simulink model "SALTStabilizationInnerOuterLoop"  (Simulink 7.8)
settings: Solver=FixedStepDiscrete  StartTime=0.0  StopTime=5.695  FixedStep=.001  RelTol=1e-3
values from neighbouring files (symbols this model uses):
  T_step = 0.01    [CoefficientsForFilters.mat]    (also in matlab.mat = 0.001)
undefined symbols (not defined in the file or in its folder): abc, alphabeta, DiscIntNeverNeededParam, dq, MicrochipMotorControlTools, to
settings Model: Creator=root  LastModifiedBy=Pavlo
settings OptimizationCC: OptimizeModelRefInitCode=on  LifeSpan=1
settings HardwareCC: ProdBitPerInt=16  ProdBitPerPointer=16  ProdLargestAtomicInteger=Integer  ProdLargestAtomicFloat=Float  ProdIntDivRoundTo=Zero  ProdEndianess=LittleEndian  ProdWordSize=16  ProdHWDeviceType=Microchip->dsPIC
settings RTWCC: SystemTargetFile=ert.tlc  GenCodeOnly=on  TemplateMakefile=ert_default_tmf  Description=Embedded Coder  ProcessScript=ert_make_rtw_hook  RTWCompilerOptimization=On
settings CodeAppCC: IgnoreCustomStorageClasses=off
settings ERTTargetCC: MultiwordLength=2048  GenerateSampleERTMain=on  ERTCustomFileTemplate=example_file_process.tlc  ConvertIfToSwitch=off  SuppressUnreachableDefaultCases=off

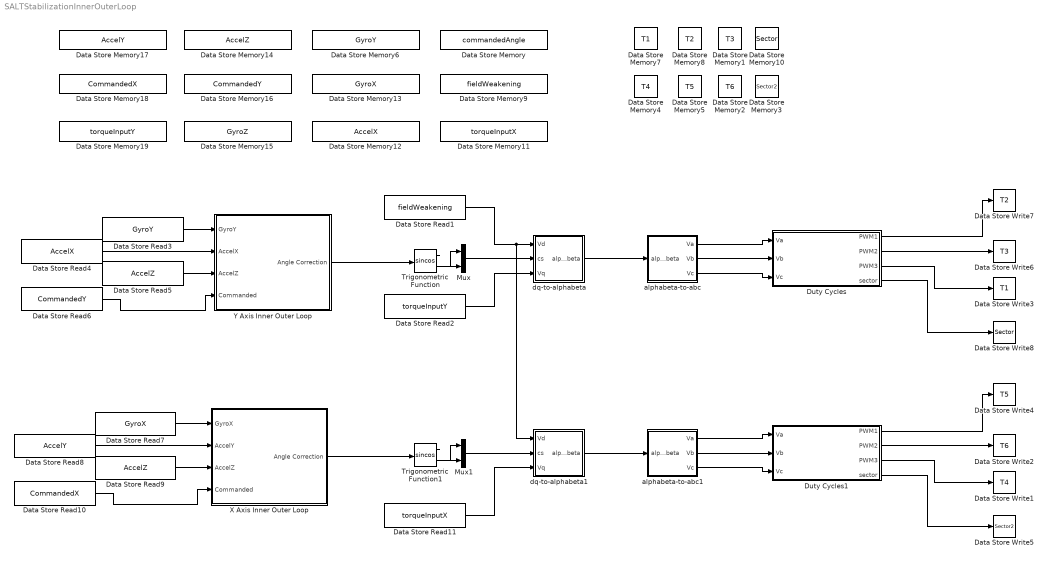
== system SALTStabilizationInnerOuterLoop ==
  Data Store Memory : DataStoreMemory  DataStoreName=commandedAngle  ReadBeforeWriteMsg=warning  WriteAfterWriteMsg=warning  WriteAfterReadMsg=warning  OutDataTypeStr=single
      settings: RTWStateStorageClass=ExportedGlobal
  Data Store Memory1 : DataStoreMemory  DataStoreName=T3  ReadBeforeWriteMsg=warning  WriteAfterWriteMsg=warning  WriteAfterReadMsg=warning  OutDataTypeStr=single
  Data Store Memory10 : DataStoreMemory  DataStoreName=Sector  ReadBeforeWriteMsg=warning  WriteAfterWriteMsg=warning  WriteAfterReadMsg=warning  OutDataTypeStr=single
  Data Store Memory11 : DataStoreMemory  DataStoreName=torqueInputX  ReadBeforeWriteMsg=warning  WriteAfterWriteMsg=warning  WriteAfterReadMsg=warning  OutDataTypeStr=single
      settings: RTWStateStorageClass=ExportedGlobal
  Data Store Memory12 : DataStoreMemory  DataStoreName=AccelX  ReadBeforeWriteMsg=warning  WriteAfterWriteMsg=warning  WriteAfterReadMsg=warning  OutDataTypeStr=single
      settings: RTWStateStorageClass=ExportedGlobal
  Data Store Memory13 : DataStoreMemory  DataStoreName=GyroX  ReadBeforeWriteMsg=warning  WriteAfterWriteMsg=warning  WriteAfterReadMsg=warning  OutDataTypeStr=single
      settings: RTWStateStorageClass=ExportedGlobal
  Data Store Memory14 : DataStoreMemory  DataStoreName=AccelZ  ReadBeforeWriteMsg=warning  WriteAfterWriteMsg=warning  WriteAfterReadMsg=warning  OutDataTypeStr=single
      settings: RTWStateStorageClass=ExportedGlobal
  Data Store Memory15 : DataStoreMemory  DataStoreName=GyroZ  ReadBeforeWriteMsg=warning  WriteAfterWriteMsg=warning  WriteAfterReadMsg=warning  OutDataTypeStr=single
      settings: RTWStateStorageClass=ExportedGlobal
  Data Store Memory16 : DataStoreMemory  DataStoreName=CommandedY  ReadBeforeWriteMsg=warning  WriteAfterWriteMsg=warning  WriteAfterReadMsg=warning  OutDataTypeStr=single
      settings: RTWStateStorageClass=ExportedGlobal
  Data Store Memory17 : DataStoreMemory  DataStoreName=AccelY  ReadBeforeWriteMsg=warning  WriteAfterWriteMsg=warning  WriteAfterReadMsg=warning  OutDataTypeStr=single
      settings: RTWStateStorageClass=ExportedGlobal
  Data Store Memory18 : DataStoreMemory  DataStoreName=CommandedX  ReadBeforeWriteMsg=warning  WriteAfterWriteMsg=warning  WriteAfterReadMsg=warning  OutDataTypeStr=single
      settings: RTWStateStorageClass=ExportedGlobal
  Data Store Memory19 : DataStoreMemory  DataStoreName=torqueInputY  ReadBeforeWriteMsg=warning  WriteAfterWriteMsg=warning  WriteAfterReadMsg=warning  OutDataTypeStr=single
      settings: RTWStateStorageClass=ExportedGlobal
  Data Store Memory2 : DataStoreMemory  DataStoreName=T6  ReadBeforeWriteMsg=warning  WriteAfterWriteMsg=warning  WriteAfterReadMsg=warning  OutDataTypeStr=single
  Data Store Memory3 : DataStoreMemory  DataStoreName=Sector2  ReadBeforeWriteMsg=warning  WriteAfterWriteMsg=warning  WriteAfterReadMsg=warning  OutDataTypeStr=single
  Data Store Memory4 : DataStoreMemory  DataStoreName=T4  ReadBeforeWriteMsg=warning  WriteAfterWriteMsg=warning  WriteAfterReadMsg=warning  OutDataTypeStr=single
  Data Store Memory5 : DataStoreMemory  DataStoreName=T5  ReadBeforeWriteMsg=warning  WriteAfterWriteMsg=warning  WriteAfterReadMsg=warning  OutDataTypeStr=single
  Data Store Memory6 : DataStoreMemory  DataStoreName=GyroY  ReadBeforeWriteMsg=warning  WriteAfterWriteMsg=warning  WriteAfterReadMsg=warning  OutDataTypeStr=single
      settings: RTWStateStorageClass=ExportedGlobal
  Data Store Memory7 : DataStoreMemory  DataStoreName=T1  ReadBeforeWriteMsg=warning  WriteAfterWriteMsg=warning  WriteAfterReadMsg=warning  OutDataTypeStr=single
  Data Store Memory8 : DataStoreMemory  DataStoreName=T2  ReadBeforeWriteMsg=warning  WriteAfterWriteMsg=warning  WriteAfterReadMsg=warning  OutDataTypeStr=single
  Data Store Memory9 : DataStoreMemory  DataStoreName=fieldWeakening  ReadBeforeWriteMsg=warning  WriteAfterWriteMsg=warning  WriteAfterReadMsg=warning  OutDataTypeStr=single
      settings: RTWStateStorageClass=ExportedGlobal
  Data Store Read1 : DataStoreRead  DataStoreName=fieldWeakening
  Data Store Read10 : DataStoreRead  DataStoreName=CommandedX
  Data Store Read11 : DataStoreRead  DataStoreName=torqueInputX
  Data Store Read2 : DataStoreRead  DataStoreName=torqueInputY
  Data Store Read3 : DataStoreRead  DataStoreName=GyroY
  Data Store Read4 : DataStoreRead  DataStoreName=AccelX
  Data Store Read5 : DataStoreRead  DataStoreName=AccelZ
  Data Store Read6 : DataStoreRead  DataStoreName=CommandedY
  Data Store Read7 : DataStoreRead  DataStoreName=GyroX
  Data Store Read8 : DataStoreRead  DataStoreName=AccelY
  Data Store Read9 : DataStoreRead  DataStoreName=AccelZ
  Data Store Write1 : DataStoreWrite  DataStoreName=T4
  Data Store Write2 : DataStoreWrite  DataStoreName=T6
  Data Store Write3 : DataStoreWrite  DataStoreName=T1
  Data Store Write4 : DataStoreWrite  DataStoreName=T5
  Data Store Write5 : DataStoreWrite  DataStoreName=Sector2
  Data Store Write6 : DataStoreWrite  DataStoreName=T3
  Data Store Write7 : DataStoreWrite  DataStoreName=T2
  Data Store Write8 : DataStoreWrite  DataStoreName=Sector
  Duty Cycles : MATLAB Function  TreatAsAtomicUnit=on
  Duty Cycles1 : MATLAB Function  TreatAsAtomicUnit=on
  Mux : Mux  Inputs=2
  Mux1 : Mux  Inputs=2
  Trigonometric Function : Trigonometry  Operator=sincos
  Trigonometric Function1 : Trigonometry  Operator=sincos
  X Axis Inner Outer Loop : Subsystem
  Y Axis Inner Outer Loop : Subsystem
  alphabeta-to-abc : Subsystem  AncestorBlock=MicrochipMotorControlTools/alphabeta-to-abc
  alphabeta-to-abc1 : Subsystem  AncestorBlock=MicrochipMotorControlTools/alphabeta-to-abc
  dq-to-alphabeta : Subsystem  AncestorBlock=MicrochipMotorControlTools/dq-to-alphabeta
  dq-to-alphabeta1 : Subsystem  AncestorBlock=MicrochipMotorControlTools/dq-to-alphabeta
  wires:
  Mux/1 -> dq-to-alphabeta/2(cs)
  dq-to-alphabeta/1(alphabeta) -> alphabeta-to-abc/1(alphabeta)
  alphabeta-to-abc/1(Va) -> Duty Cycles/1(Va)
  alphabeta-to-abc/2(Vb) -> Duty Cycles/2(Vb)
  alphabeta-to-abc/3(Vc) -> Duty Cycles/3(Vc)
  Data Store Read1/1 -> dq-to-alphabeta/1(Vd), dq-to-alphabeta1/1(Vd)
  Data Store Read2/1 -> dq-to-alphabeta/3(Vq)
  Y Axis Inner Outer Loop/1(Angle Correction) -> Trigonometric Function/1
  Duty Cycles/1(PWM1) -> Data Store Write7/1
  Duty Cycles/2(PWM2) -> Data Store Write6/1
  Duty Cycles/3(PWM3) -> Data Store Write3/1
  Duty Cycles/4(sector) -> Data Store Write8/1
  Trigonometric Function/2 -> Mux/1
  Trigonometric Function/1 -> Mux/2
  Mux1/1 -> dq-to-alphabeta1/2(cs)
  dq-to-alphabeta1/1(alphabeta) -> alphabeta-to-abc1/1(alphabeta)
  alphabeta-to-abc1/1(Va) -> Duty Cycles1/1(Va)
  alphabeta-to-abc1/2(Vb) -> Duty Cycles1/2(Vb)
  alphabeta-to-abc1/3(Vc) -> Duty Cycles1/3(Vc)
  X Axis Inner Outer Loop/1(Angle Correction) -> Trigonometric Function1/1
  Duty Cycles1/1(PWM1) -> Data Store Write4/1
  Duty Cycles1/2(PWM2) -> Data Store Write2/1
  Duty Cycles1/3(PWM3) -> Data Store Write1/1
  Duty Cycles1/4(sector) -> Data Store Write5/1
  Trigonometric Function1/2 -> Mux1/1
  Trigonometric Function1/1 -> Mux1/2
  Data Store Read3/1 -> Y Axis Inner Outer Loop/1(GyroY)
  Data Store Read4/1 -> Y Axis Inner Outer Loop/2(AccelX)
  Data Store Read5/1 -> Y Axis Inner Outer Loop/3(AccelZ)
  Data Store Read6/1 -> Y Axis Inner Outer Loop/4(Commanded)
  Data Store Read7/1 -> X Axis Inner Outer Loop/1(GyroX)
  Data Store Read8/1 -> X Axis Inner Outer Loop/2(AccelY)
  Data Store Read9/1 -> X Axis Inner Outer Loop/3(AccelZ)
  Data Store Read10/1 -> X Axis Inner Outer Loop/4(Commanded)
  Data Store Read11/1 -> dq-to-alphabeta1/3(Vq)

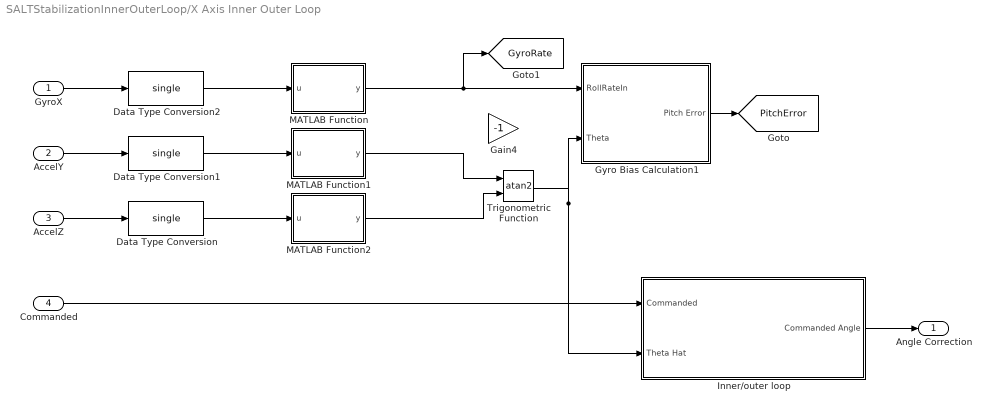
== system SALTStabilizationInnerOuterLoop/X Axis Inner Outer Loop ==
  GyroX : Inport
  AccelY : Inport  Port=2
  AccelZ : Inport  Port=3
  Commanded : Inport  Port=4
  Data Type Conversion : DataTypeConversion  OutMax=4095  OutDataTypeStr=single
  Data Type Conversion1 : DataTypeConversion  OutMax=4095  OutDataTypeStr=single
  Data Type Conversion2 : DataTypeConversion  OutMax=4095  OutDataTypeStr=single  RndMeth=Simplest
  Gain4 : Gain  Gain=-1
  Gyro Bias Calculation1 : Subsystem
  Inner/outer loop : Subsystem
  MATLAB Function : MATLAB Function  TreatAsAtomicUnit=on
  MATLAB Function1 : MATLAB Function  TreatAsAtomicUnit=on
  MATLAB Function2 : MATLAB Function  TreatAsAtomicUnit=on
  Trigonometric Function : Trigonometry  Operator=atan2
  Angle Correction : Outport
  tag scope: GyroRate=global, PitchError=global
  wires:
  AccelZ/1 -> Data Type Conversion/1
  AccelY/1 -> Data Type Conversion1/1
  GyroX/1 -> Data Type Conversion2/1
  Inner/outer loop/1(Commanded Angle) -> Angle Correction/1
  MATLAB Function2/1(y) -> Trigonometric Function/2
  MATLAB Function1/1(y) -> Trigonometric Function/1
  MATLAB Function/1(y) -> [GyroRate], Gyro Bias Calculation1/1(RollRateIn)
  Data Type Conversion/1 -> MATLAB Function2/1(u)
  Data Type Conversion1/1 -> MATLAB Function1/1(u)
  Trigonometric Function/1 -> Gyro Bias Calculation1/2(Theta), Inner/outer loop/2(Theta Hat)
  Data Type Conversion2/1 -> MATLAB Function/1(u)
  Gyro Bias Calculation1/1(Pitch Error) -> [PitchError]
  Commanded/1 -> Inner/outer loop/1(Commanded)

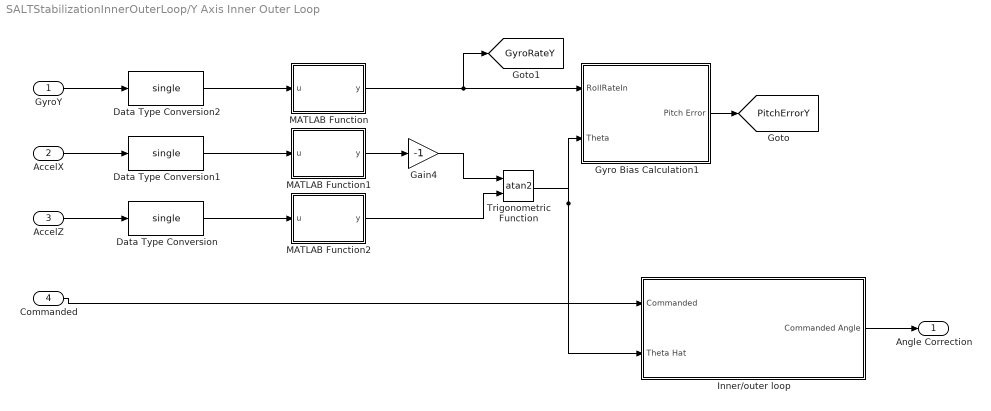
== system SALTStabilizationInnerOuterLoop/Y Axis Inner Outer Loop ==
  GyroY : Inport
  AccelX : Inport  Port=2
  AccelZ : Inport  Port=3
  Commanded : Inport  Port=4
  Data Type Conversion : DataTypeConversion  OutMax=4095  OutDataTypeStr=single
  Data Type Conversion1 : DataTypeConversion  OutMax=4095  OutDataTypeStr=single
  Data Type Conversion2 : DataTypeConversion  OutMax=4095  OutDataTypeStr=single  RndMeth=Simplest
  Gain4 : Gain  Gain=-1
  Gyro Bias Calculation1 : Subsystem
  Inner/outer loop : Subsystem
  MATLAB Function : MATLAB Function  TreatAsAtomicUnit=on
  MATLAB Function1 : MATLAB Function  TreatAsAtomicUnit=on
  MATLAB Function2 : MATLAB Function  TreatAsAtomicUnit=on
  Trigonometric Function : Trigonometry  Operator=atan2
  Angle Correction : Outport
  tag scope: GyroRateY=global, PitchErrorY=global
  wires:
  AccelZ/1 -> Data Type Conversion/1
  AccelX/1 -> Data Type Conversion1/1
  GyroY/1 -> Data Type Conversion2/1
  Inner/outer loop/1(Commanded Angle) -> Angle Correction/1
  Gain4/1 -> Trigonometric Function/1
  MATLAB Function2/1(y) -> Trigonometric Function/2
  MATLAB Function1/1(y) -> Gain4/1
  MATLAB Function/1(y) -> [GyroRateY], Gyro Bias Calculation1/1(RollRateIn)
  Data Type Conversion/1 -> MATLAB Function2/1(u)
  Data Type Conversion1/1 -> MATLAB Function1/1(u)
  Trigonometric Function/1 -> Gyro Bias Calculation1/2(Theta), Inner/outer loop/2(Theta Hat)
  Data Type Conversion2/1 -> MATLAB Function/1(u)
  Gyro Bias Calculation1/1(Pitch Error) -> [PitchErrorY]
  Commanded/1 -> Inner/outer loop/1(Commanded)

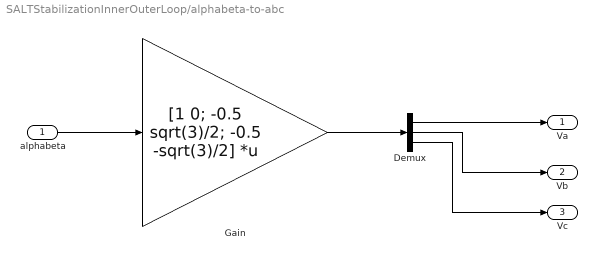
== system SALTStabilizationInnerOuterLoop/alphabeta-to-abc ==
  alphabeta : Inport
  Demux : Demux  Outputs=3
  Gain : Gain  Gain=[1 0; -0.5 sqrt(3)/2; -0.5 -sqrt(3)/2]  Multiplication=Matrix(K*u)  OutDataTypeStr=single
  Va : Outport  OutDataTypeStr=single
  Vb : Outport  Port=2  OutDataTypeStr=single
  Vc : Outport  Port=3  OutDataTypeStr=single
  wires:
  alphabeta/1 -> Gain/1
  Gain/1 -> Demux/1
  Demux/1 -> Va/1
  Demux/2 -> Vb/1
  Demux/3 -> Vc/1

== system SALTStabilizationInnerOuterLoop/alphabeta-to-abc1 ==
  alphabeta : Inport
  Demux : Demux  Outputs=3
  Gain : Gain  Gain=[1 0; -0.5 sqrt(3)/2; -0.5 -sqrt(3)/2]  Multiplication=Matrix(K*u)  OutDataTypeStr=single
  Va : Outport  OutDataTypeStr=single
  Vb : Outport  Port=2  OutDataTypeStr=single
  Vc : Outport  Port=3  OutDataTypeStr=single
  wires:
  alphabeta/1 -> Gain/1
  Gain/1 -> Demux/1
  Demux/1 -> Va/1
  Demux/2 -> Vb/1
  Demux/3 -> Vc/1

== system SALTStabilizationInnerOuterLoop/dq-to-alphabeta ==
  Vd : Inport
  cs : Inport  Port=2
  Vq : Inport  Port=3
  vector mixer : Subsystem  AncestorBlock=MicrochipMotorControlTools/vector mixer
  alphabeta : Outport
  wires:
  cs/1 -> vector mixer/2(B)
  Vd/1 -> vector mixer/1(Ax)
  vector mixer/1(C) -> alphabeta/1
  Vq/1 -> vector mixer/3(Ay)

== system SALTStabilizationInnerOuterLoop/dq-to-alphabeta1 ==
  Vd : Inport
  cs : Inport  Port=2
  Vq : Inport  Port=3
  vector mixer : Subsystem  AncestorBlock=MicrochipMotorControlTools/vector mixer
  alphabeta : Outport
  wires:
  cs/1 -> vector mixer/2(B)
  Vd/1 -> vector mixer/1(Ax)
  vector mixer/1(C) -> alphabeta/1
  Vq/1 -> vector mixer/3(Ay)

== system SALTStabilizationInnerOuterLoop/X Axis Inner Outer Loop/Gyro Bias Calculation1 ==
  RollRateIn : Inport
  Theta : Inport  Port=2
  Add : Sum  Inputs=+-
  Discrete-Time Integrator : DiscreteIntegrator  IntegratorMethod=Integration: Trapezoidal  SampleTime=T_step  UpperSaturationLimit=1  LowerSaturationLimit=-1  ICPrevOutput=DiscIntNeverNeededParam  ICPrevScaledInput=DiscIntNeverNeededParam
  Pitch Error : Outport
  wires:
  RollRateIn/1 -> Discrete-Time Integrator/1
  Add/1 -> Pitch Error/1
  Discrete-Time Integrator/1 -> Add/1
  Theta/1 -> Add/2

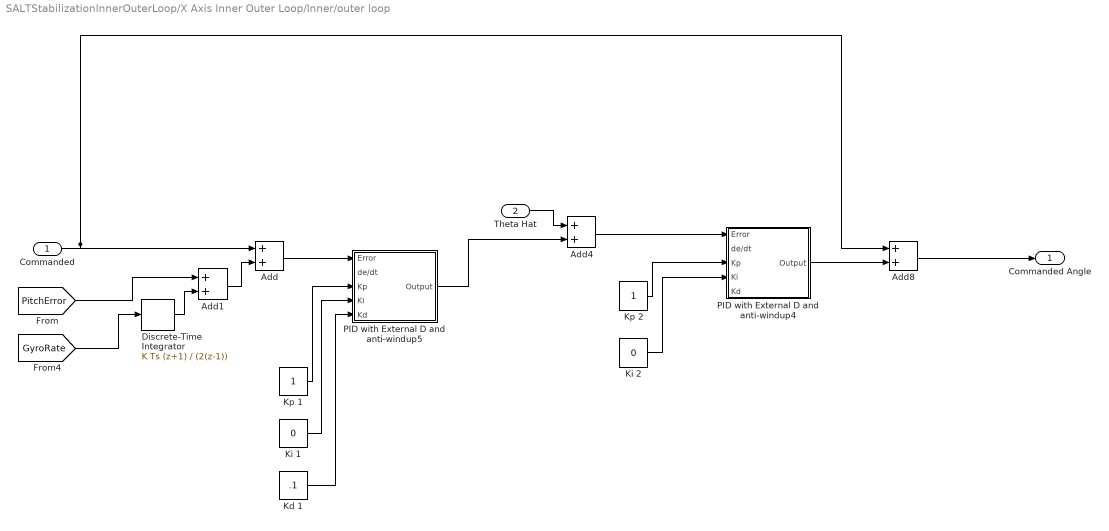
== system SALTStabilizationInnerOuterLoop/X Axis Inner Outer Loop/Inner/outer loop ==
  Commanded : Inport
  Theta Hat : Inport  Port=2
  Add{,1,4,8} (4 alike) : Sum
  Discrete-Time Integrator : DiscreteIntegrator  IntegratorMethod=Integration: Trapezoidal  SampleTime=T_step  ICPrevOutput=DiscIntNeverNeededParam  ICPrevScaledInput=DiscIntNeverNeededParam
  Kd 1 : Constant  Value=.1
  Ki 1 : Constant  Value=0
  Ki 2 : Constant  Value=0
  Kp 1 : Constant
  Kp 2 : Constant
  PID with External D and anti-windup4 : Subsystem
  PID with External D and anti-windup5 : Subsystem
  Commanded Angle : Outport
  wires:
  Add8/1 -> Commanded Angle/1
  Commanded/1 -> Add8/1, Add/1
  Kp 1/1 -> PID with External D and anti-windup5/3(Kp)
  Ki 1/1 -> PID with External D and anti-windup5/4(Ki)
  Kd 1/1 -> PID with External D and anti-windup5/5(Kd)
  Add4/1 -> PID with External D and anti-windup4/1(Error)
  Kp 2/1 -> PID with External D and anti-windup4/3(Kp)
  Ki 2/1 -> PID with External D and anti-windup4/4(Ki)
  [GyroRate] -> Discrete-Time Integrator/1
  Theta Hat/1 -> Add4/1
  PID with External D and anti-windup4/1(Output) -> Add8/2
  Add/1 -> PID with External D and anti-windup5/1(Error)
  PID with External D and anti-windup5/1(Output) -> Add4/2
  Add1/1 -> Add/2
  Discrete-Time Integrator/1 -> Add1/2
  [PitchError] -> Add1/1

== system SALTStabilizationInnerOuterLoop/Y Axis Inner Outer Loop/Gyro Bias Calculation1 ==
  RollRateIn : Inport
  Theta : Inport  Port=2
  Add : Sum  Inputs=+-
  Discrete-Time Integrator : DiscreteIntegrator  IntegratorMethod=Integration: Trapezoidal  SampleTime=T_step  UpperSaturationLimit=1  LowerSaturationLimit=-1  ICPrevOutput=DiscIntNeverNeededParam  ICPrevScaledInput=DiscIntNeverNeededParam
  Pitch Error : Outport
  wires:
  RollRateIn/1 -> Discrete-Time Integrator/1
  Add/1 -> Pitch Error/1
  Discrete-Time Integrator/1 -> Add/1
  Theta/1 -> Add/2

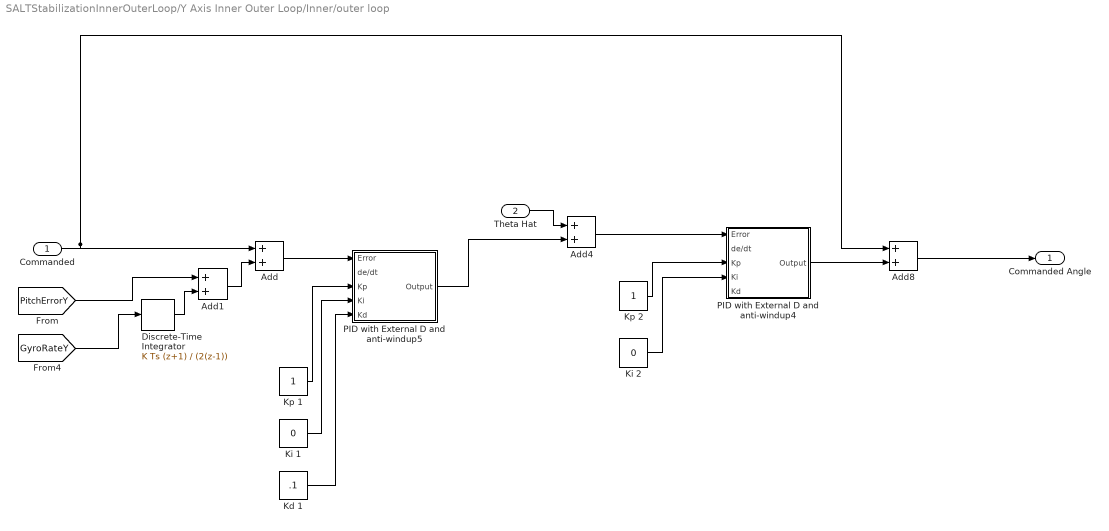
== system SALTStabilizationInnerOuterLoop/Y Axis Inner Outer Loop/Inner/outer loop ==
  Commanded : Inport
  Theta Hat : Inport  Port=2
  Add{,1,4,8} (4 alike) : Sum
  Discrete-Time Integrator : DiscreteIntegrator  IntegratorMethod=Integration: Trapezoidal  SampleTime=T_step  ICPrevOutput=DiscIntNeverNeededParam  ICPrevScaledInput=DiscIntNeverNeededParam
  Kd 1 : Constant  Value=.1
  Ki 1 : Constant  Value=0
  Ki 2 : Constant  Value=0
  Kp 1 : Constant
  Kp 2 : Constant
  PID with External D and anti-windup4 : Subsystem
  PID with External D and anti-windup5 : Subsystem
  Commanded Angle : Outport
  wires:
  Add8/1 -> Commanded Angle/1
  Commanded/1 -> Add8/1, Add/1
  Kp 1/1 -> PID with External D and anti-windup5/3(Kp)
  Ki 1/1 -> PID with External D and anti-windup5/4(Ki)
  Kd 1/1 -> PID with External D and anti-windup5/5(Kd)
  Add4/1 -> PID with External D and anti-windup4/1(Error)
  Kp 2/1 -> PID with External D and anti-windup4/3(Kp)
  Ki 2/1 -> PID with External D and anti-windup4/4(Ki)
  [GyroRateY] -> Discrete-Time Integrator/1
  Theta Hat/1 -> Add4/1
  PID with External D and anti-windup4/1(Output) -> Add8/2
  Add/1 -> PID with External D and anti-windup5/1(Error)
  PID with External D and anti-windup5/1(Output) -> Add4/2
  Add1/1 -> Add/2
  Discrete-Time Integrator/1 -> Add1/2
  [PitchErrorY] -> Add1/1

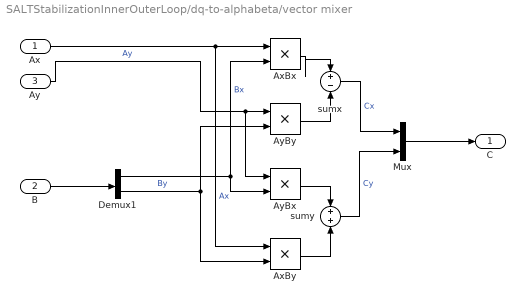
== system SALTStabilizationInnerOuterLoop/dq-to-alphabeta/vector mixer ==
  Ax : Inport
  B : Inport  Port=2
  Ay : Inport  Port=3
  AxBx : Product  RndMeth=Zero  OutDataTypeStr=Inherit: Same as first input
  AxBy : Product  RndMeth=Zero  OutDataTypeStr=Inherit: Same as first input
  AyBx : Product  RndMeth=Zero  OutDataTypeStr=Inherit: Same as first input
  AyBy : Product  RndMeth=Zero  OutDataTypeStr=Inherit: Same as first input
  Demux1 : Demux  Outputs=2
  Mux : Mux  Inputs=2
  sumx : Sum  Inputs=+|-
  sumy : Sum  Inputs=+|+
  C : Outport
  wires:
  sumx/1 -> Mux/1  "Cx"
  B/1 -> Demux1/1
  Demux1/1 -> AyBx/2, AxBx/2  "Bx"
  Demux1/2 -> AxBy/2, AyBy/2  "By"
  sumy/1 -> Mux/2  "Cy"
  AxBy/1 -> sumy/2
  AyBx/1 -> sumy/1
  AxBx/1 -> sumx/1
  AyBy/1 -> sumx/2
  Ay/1 -> AyBy/1, AyBx/1  "Ay"
  Ax/1 -> AxBy/1, AxBx/1  "Ax"
  Mux/1 -> C/1

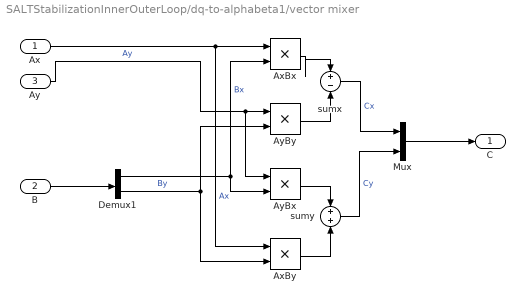
== system SALTStabilizationInnerOuterLoop/dq-to-alphabeta1/vector mixer ==
  Ax : Inport
  B : Inport  Port=2
  Ay : Inport  Port=3
  AxBx : Product  RndMeth=Zero  OutDataTypeStr=Inherit: Same as first input
  AxBy : Product  RndMeth=Zero  OutDataTypeStr=Inherit: Same as first input
  AyBx : Product  RndMeth=Zero  OutDataTypeStr=Inherit: Same as first input
  AyBy : Product  RndMeth=Zero  OutDataTypeStr=Inherit: Same as first input
  Demux1 : Demux  Outputs=2
  Mux : Mux  Inputs=2
  sumx : Sum  Inputs=+|-
  sumy : Sum  Inputs=+|+
  C : Outport
  wires:
  sumx/1 -> Mux/1  "Cx"
  B/1 -> Demux1/1
  Demux1/1 -> AyBx/2, AxBx/2  "Bx"
  Demux1/2 -> AxBy/2, AyBy/2  "By"
  sumy/1 -> Mux/2  "Cy"
  AxBy/1 -> sumy/2
  AyBx/1 -> sumy/1
  AxBx/1 -> sumx/1
  AyBy/1 -> sumx/2
  Ay/1 -> AyBy/1, AyBx/1  "Ay"
  Ax/1 -> AxBy/1, AxBx/1  "Ax"
  Mux/1 -> C/1

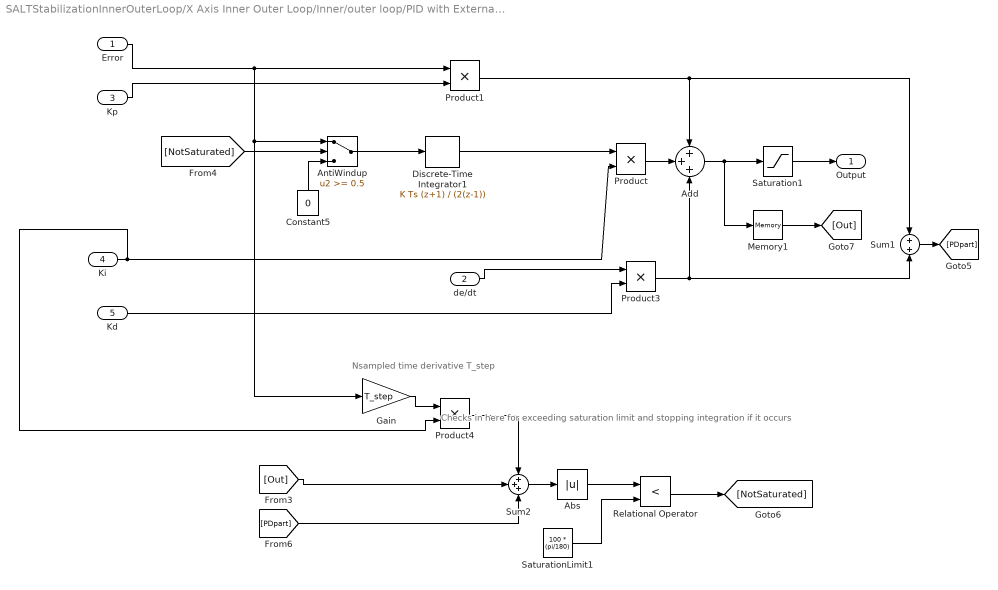
== system SALTStabilizationInnerOuterLoop/X Axis Inner Outer Loop/Inner/outer loop/PID with External D and anti-windup4 ==
  note: Nsampled time derivative
      | T_step
  note: Checks in here for
      | exceeding saturation
      | limit and stopping
      | integration if it occurs
  Error : Inport
  de/dt : Inport  Port=2
  Kp : Inport  Port=3
  Ki : Inport  Port=4
  Kd : Inport  Port=5
  Abs : Abs
  Add : Sum  Inputs=+++
  AntiWindup : Switch  Threshold=0.5
  Constant5 : Constant  Value=0  OutDataTypeStr=double
  Discrete-Time Integrator1 : DiscreteIntegrator  IntegratorMethod=Integration: Trapezoidal  SampleTime=T_step  ICPrevOutput=DiscIntNeverNeededParam  ICPrevScaledInput=DiscIntNeverNeededParam
  Gain : Gain  Gain=T_step
  Memory1 : Memory  InheritSampleTime=on
  Product{,1,3..4} (4 alike) : Product  RndMeth=Zero
  Relational Operator : RelationalOperator  Operator=<  OutDataTypeStr=boolean
  Saturation1 : Saturate  UpperLimit=pi  LowerLimit=-pi
  SaturationLimit1 : Constant  Value=100 * (pi/180)
  Sum1 : Sum  Inputs=+|+
  Sum2 : Sum  Inputs=+++
  Output : Outport
  wires:
  [NotSaturated] -> AntiWindup/2
  Abs/1 -> Relational Operator/1
  SaturationLimit1/1 -> Relational Operator/2
  Saturation1/1 -> Output/1
  Product3/1 -> Add/3, Sum1/2
  de/dt/1 -> Product3/1
  Kd/1 -> Product3/2
  Add/1 -> Memory1/1, Saturation1/1
  Product1/1 -> Sum1/1, Add/1
  Product/1 -> Add/2
  Kp/1 -> Product1/2
  Discrete-Time Integrator1/1 -> Product/1
  Ki/1 -> Product/2, Product4/2
  Error/1 -> Product1/1, AntiWindup/1, Gain/1
  AntiWindup/1 -> Discrete-Time Integrator1/1
  Constant5/1 -> AntiWindup/3
  Sum1/1 -> [PDpart]
  [Out] -> Sum2/2
  Sum2/1 -> Abs/1
  Gain/1 -> Product4/1
  Product4/1 -> Sum2/1
  Memory1/1 -> [Out]
  [PDpart] -> Sum2/3
  Relational Operator/1 -> [NotSaturated]

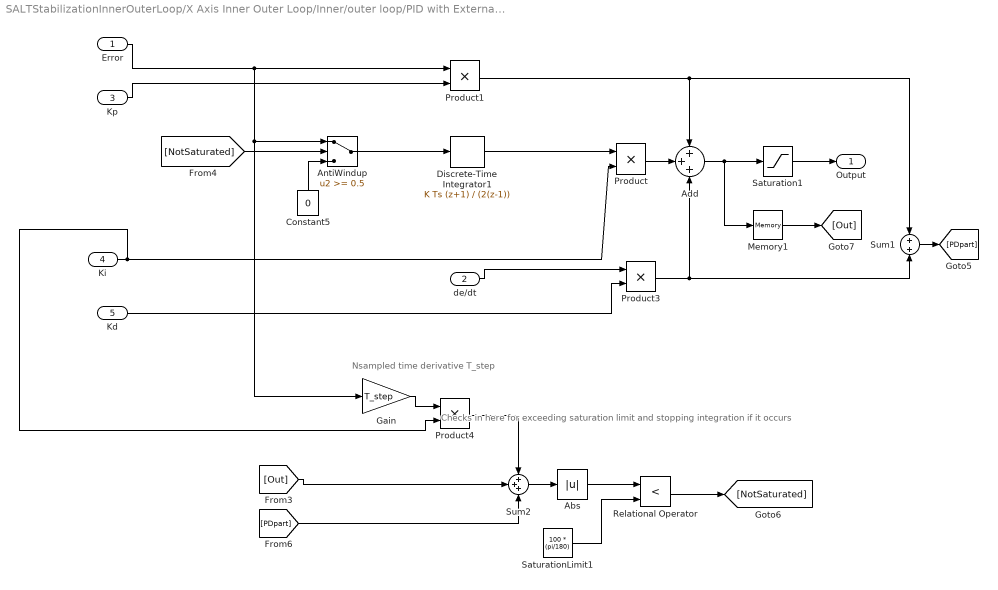
== system SALTStabilizationInnerOuterLoop/X Axis Inner Outer Loop/Inner/outer loop/PID with External D and anti-windup5 ==
  note: Nsampled time derivative
      | T_step
  note: Checks in here for
      | exceeding saturation
      | limit and stopping
      | integration if it occurs
  Error : Inport
  de/dt : Inport  Port=2
  Kp : Inport  Port=3
  Ki : Inport  Port=4
  Kd : Inport  Port=5
  Abs : Abs
  Add : Sum  Inputs=+++
  AntiWindup : Switch  Threshold=0.5
  Constant5 : Constant  Value=0  OutDataTypeStr=double
  Discrete-Time Integrator1 : DiscreteIntegrator  IntegratorMethod=Integration: Trapezoidal  SampleTime=T_step  ICPrevOutput=DiscIntNeverNeededParam  ICPrevScaledInput=DiscIntNeverNeededParam
  Gain : Gain  Gain=T_step
  Memory1 : Memory  InheritSampleTime=on
  Product{,1,3..4} (4 alike) : Product  RndMeth=Zero
  Relational Operator : RelationalOperator  Operator=<  OutDataTypeStr=boolean
  Saturation1 : Saturate  UpperLimit=pi  LowerLimit=-pi
  SaturationLimit1 : Constant  Value=100 * (pi/180)
  Sum1 : Sum  Inputs=+|+
  Sum2 : Sum  Inputs=+++
  Output : Outport
  wires:
  [NotSaturated] -> AntiWindup/2
  Abs/1 -> Relational Operator/1
  SaturationLimit1/1 -> Relational Operator/2
  Saturation1/1 -> Output/1
  Product3/1 -> Add/3, Sum1/2
  de/dt/1 -> Product3/1
  Kd/1 -> Product3/2
  Add/1 -> Memory1/1, Saturation1/1
  Product1/1 -> Sum1/1, Add/1
  Product/1 -> Add/2
  Kp/1 -> Product1/2
  Discrete-Time Integrator1/1 -> Product/1
  Ki/1 -> Product/2, Product4/2
  Error/1 -> Product1/1, AntiWindup/1, Gain/1
  AntiWindup/1 -> Discrete-Time Integrator1/1
  Constant5/1 -> AntiWindup/3
  Sum1/1 -> [PDpart]
  [Out] -> Sum2/2
  Sum2/1 -> Abs/1
  Gain/1 -> Product4/1
  Product4/1 -> Sum2/1
  Memory1/1 -> [Out]
  [PDpart] -> Sum2/3
  Relational Operator/1 -> [NotSaturated]

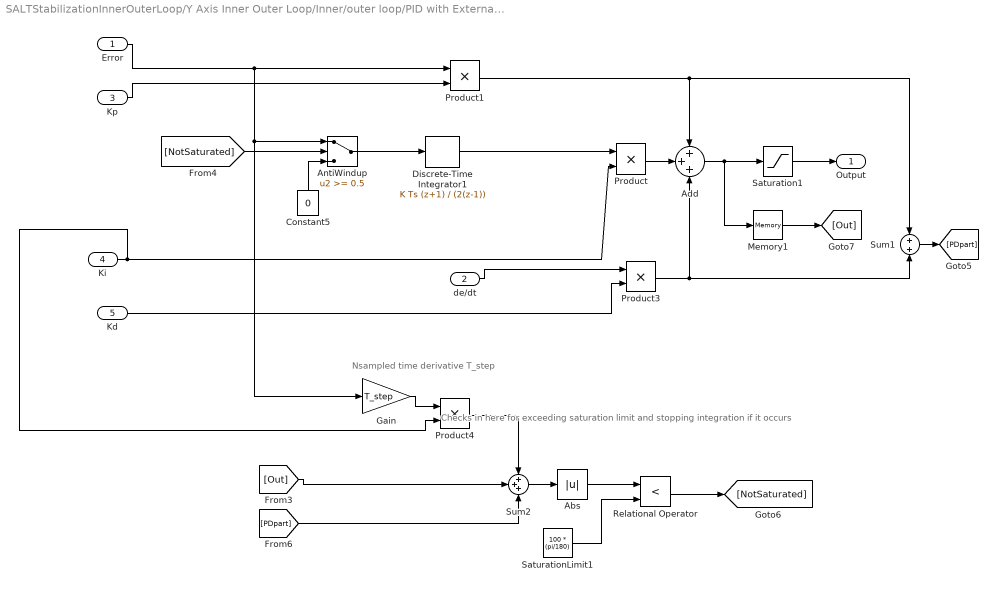
== system SALTStabilizationInnerOuterLoop/Y Axis Inner Outer Loop/Inner/outer loop/PID with External D and anti-windup4 ==
  note: Nsampled time derivative
      | T_step
  note: Checks in here for
      | exceeding saturation
      | limit and stopping
      | integration if it occurs
  Error : Inport
  de/dt : Inport  Port=2
  Kp : Inport  Port=3
  Ki : Inport  Port=4
  Kd : Inport  Port=5
  Abs : Abs
  Add : Sum  Inputs=+++
  AntiWindup : Switch  Threshold=0.5
  Constant5 : Constant  Value=0  OutDataTypeStr=double
  Discrete-Time Integrator1 : DiscreteIntegrator  IntegratorMethod=Integration: Trapezoidal  SampleTime=T_step  ICPrevOutput=DiscIntNeverNeededParam  ICPrevScaledInput=DiscIntNeverNeededParam
  Gain : Gain  Gain=T_step
  Memory1 : Memory  InheritSampleTime=on
  Product{,1,3..4} (4 alike) : Product  RndMeth=Zero
  Relational Operator : RelationalOperator  Operator=<  OutDataTypeStr=boolean
  Saturation1 : Saturate  UpperLimit=pi  LowerLimit=-pi
  SaturationLimit1 : Constant  Value=100 * (pi/180)
  Sum1 : Sum  Inputs=+|+
  Sum2 : Sum  Inputs=+++
  Output : Outport
  wires:
  [NotSaturated] -> AntiWindup/2
  Abs/1 -> Relational Operator/1
  SaturationLimit1/1 -> Relational Operator/2
  Saturation1/1 -> Output/1
  Product3/1 -> Add/3, Sum1/2
  de/dt/1 -> Product3/1
  Kd/1 -> Product3/2
  Add/1 -> Memory1/1, Saturation1/1
  Product1/1 -> Sum1/1, Add/1
  Product/1 -> Add/2
  Kp/1 -> Product1/2
  Discrete-Time Integrator1/1 -> Product/1
  Ki/1 -> Product/2, Product4/2
  Error/1 -> Product1/1, AntiWindup/1, Gain/1
  AntiWindup/1 -> Discrete-Time Integrator1/1
  Constant5/1 -> AntiWindup/3
  Sum1/1 -> [PDpart]
  [Out] -> Sum2/2
  Sum2/1 -> Abs/1
  Gain/1 -> Product4/1
  Product4/1 -> Sum2/1
  Memory1/1 -> [Out]
  [PDpart] -> Sum2/3
  Relational Operator/1 -> [NotSaturated]

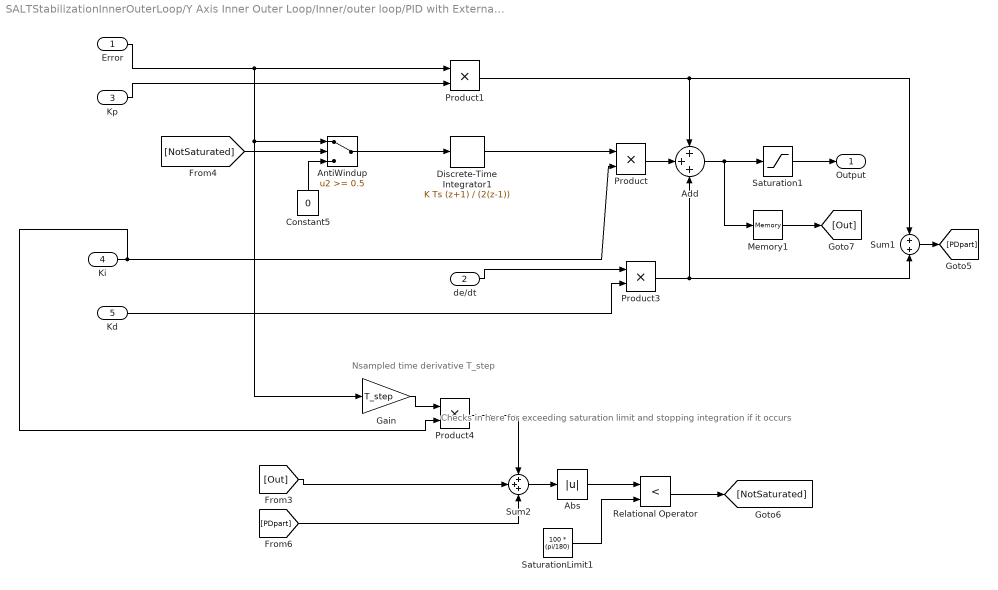
== system SALTStabilizationInnerOuterLoop/Y Axis Inner Outer Loop/Inner/outer loop/PID with External D and anti-windup5 ==
  note: Nsampled time derivative
      | T_step
  note: Checks in here for
      | exceeding saturation
      | limit and stopping
      | integration if it occurs
  Error : Inport
  de/dt : Inport  Port=2
  Kp : Inport  Port=3
  Ki : Inport  Port=4
  Kd : Inport  Port=5
  Abs : Abs
  Add : Sum  Inputs=+++
  AntiWindup : Switch  Threshold=0.5
  Constant5 : Constant  Value=0  OutDataTypeStr=double
  Discrete-Time Integrator1 : DiscreteIntegrator  IntegratorMethod=Integration: Trapezoidal  SampleTime=T_step  ICPrevOutput=DiscIntNeverNeededParam  ICPrevScaledInput=DiscIntNeverNeededParam
  Gain : Gain  Gain=T_step
  Memory1 : Memory  InheritSampleTime=on
  Product{,1,3..4} (4 alike) : Product  RndMeth=Zero
  Relational Operator : RelationalOperator  Operator=<  OutDataTypeStr=boolean
  Saturation1 : Saturate  UpperLimit=pi  LowerLimit=-pi
  SaturationLimit1 : Constant  Value=100 * (pi/180)
  Sum1 : Sum  Inputs=+|+
  Sum2 : Sum  Inputs=+++
  Output : Outport
  wires:
  [NotSaturated] -> AntiWindup/2
  Abs/1 -> Relational Operator/1
  SaturationLimit1/1 -> Relational Operator/2
  Saturation1/1 -> Output/1
  Product3/1 -> Add/3, Sum1/2
  de/dt/1 -> Product3/1
  Kd/1 -> Product3/2
  Add/1 -> Memory1/1, Saturation1/1
  Product1/1 -> Sum1/1, Add/1
  Product/1 -> Add/2
  Kp/1 -> Product1/2
  Discrete-Time Integrator1/1 -> Product/1
  Ki/1 -> Product/2, Product4/2
  Error/1 -> Product1/1, AntiWindup/1, Gain/1
  AntiWindup/1 -> Discrete-Time Integrator1/1
  Constant5/1 -> AntiWindup/3
  Sum1/1 -> [PDpart]
  [Out] -> Sum2/2
  Sum2/1 -> Abs/1
  Gain/1 -> Product4/1
  Product4/1 -> Sum2/1
  Memory1/1 -> [Out]
  [PDpart] -> Sum2/3
  Relational Operator/1 -> [NotSaturated]

== matlab function Y Axis Inner Outer Loop/MATLAB Function1 ==
  data: u input double; y output double
function y = fcn(u)
%#codegen

y = u/32.8;

== matlab function Y Axis Inner Outer Loop/MATLAB Function ==
  data: u input double; y output double
function y = fcn(u)
%#codegen

y = ((u/131) * (pi/180))*5;

== matlab function Y Axis Inner Outer Loop/MATLAB Function2 ==
  data: u input double; y output double
function y = fcn(u)
%#codegen

y = u/32.8;

== matlab function X Axis Inner Outer Loop/MATLAB Function ==
  data: u input double; y output double
function y = fcn(u)
%#codegen

y = ((u/131) * (pi/180))*5;

== matlab function X Axis Inner Outer Loop/MATLAB Function1 ==
  data: u input double; y output double
function y = fcn(u)
%#codegen

y = u/32.8;

== matlab function X Axis Inner Outer Loop/MATLAB Function2 ==
  data: u input double; y output double
function y = fcn(u)
%#codegen

y = u/32.8;

== matlab function Duty Cycles ==
  data: PWM1 output single; Va input single; PWM2 output single; PWM3 output single; sector output double; Vb input double; Vc input double
function [PWM1, PWM2, PWM3, sector]  = DutyCycleCalc(Va, Vb, Vc)
%#codegen
PWM = single(100);

Ta = single(0);

if (Va >= 0)
    if (Vb >= 0)
        %Sector 3, 0 - 60 Degrees
        T1 = Vb;
        T2 = Va;
    
        T1 = T1*PWM;
        T2 = T2*PWM;
        Tc = (PWM-T1-T2)/2;
        Tb = Ta + T1;
        Ta = Tb + T2;
    
        PWM1 = single(0);
        PWM2 = Tb;
        PWM3 = Ta;
        sector = single(3);
    else
        if (Vc >= 0)
           %Sector 5, 120 - 180 Degrees
            T1 = Va;
            T2 = Vc;
    
            T1 = T1*PWM;
            T2 = T2*PWM;
            Tc = (PWM-T1-T2)/2;
            Tb = Ta + T1;
            Ta = Tb + T2;
    
            PWM1 = Ta;
            PWM2 = single(0);
            PWM3 = Tb;
            sector = single(5);
        else
            %Sector 1, 60 - 120 Degrees
            T1 = -Vb;
            T2 = -Vc;
    
            T1 = T1*PWM;
            T2 = T2*PWM;
            Tc = (PWM-T1-T2)/2;
            Tb = Ta + T1;
            Ta = Tb + T2;
    
            PWM1 = Tb;
            PWM2 = single(0);
            PWM3 = Ta;
            sector = single(1);
        end
    end
else
    if (Vb >= 0)
        if (Vc >= 0)
            %Sector 6, 240 - 300 Degrees
            T1 = Vc;
            T2 = Vb;
    
            T1 = T1*PWM;
            T2 = T2*PWM;
            Tc = (PWM-T1-T2)/2;
            Tb = Ta + T1;
            Ta = Tb + T2;
    
            PWM1 = Tb;
            PWM2 = Ta;
            PWM3 = single(0);
            sector = single(6);
        else
            %Sector 2, 300 - 0 Degrees
            T1 = -Vc;
            T2 = -Va;
    
            T1 = T1*PWM;
            T2 = T2*PWM;
            Tc = (PWM-T1-T2)/2;
            Tb = Ta + T1;
            Ta = Tb + T2;
    
            PWM1 = single(0);
            PWM2 = Ta;
            PWM3 = Tb;
            sector = single(2);
        end
    else
        %Sector 4, 180 - 240 Degrees
        T1 = -Va;
        T2 = -Vb;
    
        T1 = T1*PWM;
        T2 = T2*PWM;
        Tc = (PWM-T1-T2)/2;
        Tb = Ta + T1;
        Ta = Tb + T2;
    
        PWM1 = Ta;
        PWM2 = Tb;
        PWM3 = single(0);
        sector = single(4);
    end
end

end

== matlab function Duty Cycles1 ==
  data: PWM1 output single; Va input single; PWM2 output single; PWM3 output single; sector output double; Vb input double; Vc input double
function [PWM1, PWM2, PWM3, sector]  = DutyCycleCalc(Va, Vb, Vc)
%#codegen
PWM = single(100);

Ta = single(0);

if (Va >= 0)
    if (Vb >= 0)
        %Sector 3, 0 - 60 Degrees
        T1 = Vb;
        T2 = Va;
    
        T1 = T1*PWM;
        T2 = T2*PWM;
        Tc = (PWM-T1-T2)/2;
        Tb = Ta + T1;
        Ta = Tb + T2;
    
        PWM1 = single(0);
        PWM2 = Tb;
        PWM3 = Ta;
        sector = single(3);
    else
        if (Vc >= 0)
           %Sector 5, 120 - 180 Degrees
            T1 = Va;
            T2 = Vc;
    
            T1 = T1*PWM;
            T2 = T2*PWM;
            Tc = (PWM-T1-T2)/2;
            Tb = Ta + T1;
            Ta = Tb + T2;
    
            PWM1 = Ta;
            PWM2 = single(0);
            PWM3 = Tb;
            sector = single(5);
        else
            %Sector 1, 60 - 120 Degrees
            T1 = -Vb;
            T2 = -Vc;
    
            T1 = T1*PWM;
            T2 = T2*PWM;
            Tc = (PWM-T1-T2)/2;
            Tb = Ta + T1;
            Ta = Tb + T2;
    
            PWM1 = Tb;
            PWM2 = single(0);
            PWM3 = Ta;
            sector = single(1);
        end
    end
else
    if (Vb >= 0)
        if (Vc >= 0)
            %Sector 6, 240 - 300 Degrees
            T1 = Vc;
            T2 = Vb;
    
            T1 = T1*PWM;
            T2 = T2*PWM;
            Tc = (PWM-T1-T2)/2;
            Tb = Ta + T1;
            Ta = Tb + T2;
    
            PWM1 = Tb;
            PWM2 = Ta;
            PWM3 = single(0);
            sector = single(6);
        else
            %Sector 2, 300 - 0 Degrees
            T1 = -Vc;
            T2 = -Va;
    
            T1 = T1*PWM;
            T2 = T2*PWM;
            Tc = (PWM-T1-T2)/2;
            Tb = Ta + T1;
            Ta = Tb + T2;
    
            PWM1 = single(0);
            PWM2 = Ta;
            PWM3 = Tb;
            sector = single(2);
        end
    else
        %Sector 4, 180 - 240 Degrees
        T1 = -Va;
        T2 = -Vb;
    
        T1 = T1*PWM;
        T2 = T2*PWM;
        Tc = (PWM-T1-T2)/2;
        Tb = Ta + T1;
        Ta = Tb + T2;
    
        PWM1 = Ta;
        PWM2 = Tb;
        PWM3 = single(0);
        sector = single(4);
    end
end

end
